simulink library "pbnbs"  (Simulink 8.1)
settings: Solver=ode1  StartTime=0.0  StopTime=Inf  FixedStep=0.001  RelTol=1e-3
PostLoadFcn:
  | , if any(exist('dsrtsu_mdlpostloadfcn', 'file') == [2, 3, 6]), try dsrtsu_mdlpostloadfcn('Execute', bdroot); catch fprintf('Error in PostLoadFcn (dsrtsu_mdlpostloadfcn) for model "%s":\n %s\n', bdroot, lasterr); end, end,
libraries: ebdc x1, frdc x1
settings Model: DSRTSU_INTERNAL_RTI_VER=450  DSRTSU_INTERNAL_RTI_TYPE=rti1401  RTICANMMDATA=struct('GeneralSetupData',struct('modelroot','D:\ELN150201_TAIWAN\trunk\AdasDragon\software\sw_development\arch\app\jud','generalsettings',struct('filesettings',struct('destfolder',struct('Name','RTICANMM_FILES','Check',1),'buildfolder',struct('Name','.','Check',1),'AbsDestfolder',struct('Name','D:\ELN150201_TAIWAN\trunk\AdasDragon\software\sw_development\arch\app\jud\RTICANMM_FILES'),'AbsBuildfolder',struct('Name','D:\ELN150201_TAIWAN\trunk\AdasDragon\software\sw_development\arch\app\jud'))),'options',struct('addpaths',1,'rmpaths',1,'addtrcexclusion',logical(1),'cannavigator',struct('checkmonitoring',0),'show_usrtrc',0,'use_usrtrc',0),'advanced',struct('options',[1 1 1 1 1 1 1 1 1 1 1 1 1 1 1 1 1 1 1 1 1 1 1 1 1 1 1 1 1 1 1 1 1 1 1 1 1 1 1 1 1 1 1 1 1 1 1 1 1 1 1 1 1 1 1 1 1 1 1 1 1 1 1 1 1 1 1 1 1 1 1 1 1 1 1 1 1 1 1 1 1 1 1 1 1 1 1 1 1 1 1 1 1 1 1 1 1 1 1 1]),'MPSetup',{{}},'modelname','pbnbs','block','pbnbs'))  DSRTSU_INTERNAL_RTIFPGA=40  Creator=tescamilla  LastModifiedBy=AT015555

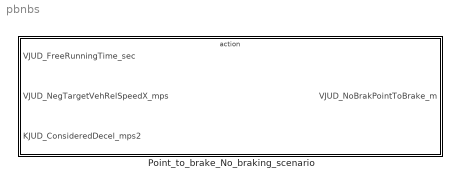
== system pbnbs ==
  Point_to_brake_No_braking_scenario : Subsystem

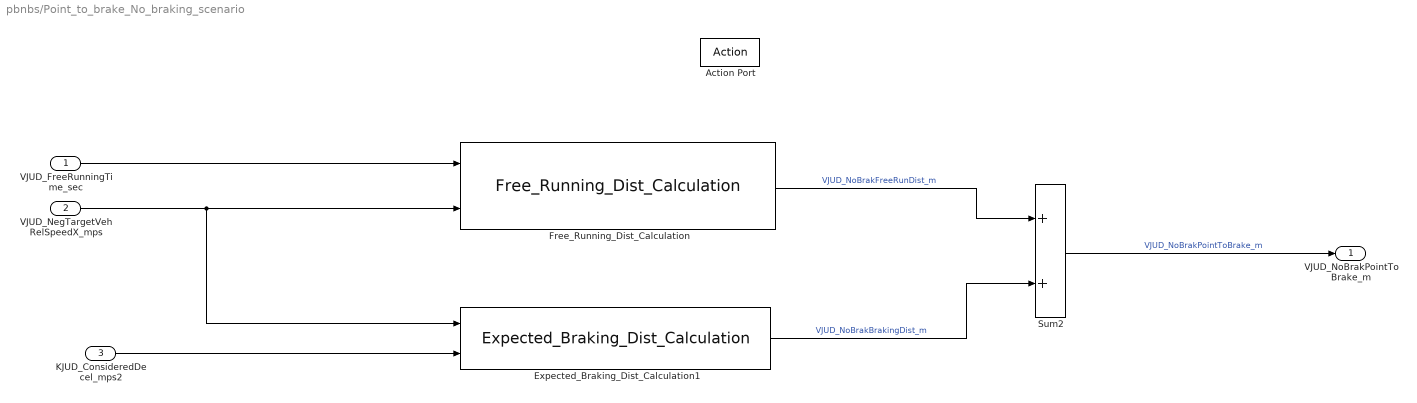
== system pbnbs/Point_to_brake_No_braking_scenario ==
  VJUD_FreeRunningTime_sec : Inport
  VJUD_NegTargetVehRelSpeedX_mps : Inport  Port=2
  KJUD_ConsideredDecel_mps2 : Inport  Port=3
  Action Port : ActionPort
  Expected_Braking_Dist_Calculation1 : ebdc/Expected_Braking_Dist_Calculation
  Free_Running_Dist_Calculation : frdc/Free_Running_Dist_Calculation
  Sum2 : Sum
  VJUD_NoBrakPointToBrake_m : Outport
  wires:
  VJUD_FreeRunningTime_sec/1 -> Free_Running_Dist_Calculation/1
  Sum2/1 -> VJUD_NoBrakPointToBrake_m/1  "VJUD_NoBrakPointToBrake_m"
  Expected_Braking_Dist_Calculation1/1 -> Sum2/2  "VJUD_NoBrakBrakingDist_m"
  KJUD_ConsideredDecel_mps2/1 -> Expected_Braking_Dist_Calculation1/2
  Free_Running_Dist_Calculation/1 -> Sum2/1  "VJUD_NoBrakFreeRunDist_m"
  VJUD_NegTargetVehRelSpeedX_mps/1 -> Free_Running_Dist_Calculation/2, Expected_Braking_Dist_Calculation1/1
